simulink model "ITSC2021_CoupledPathFollowingSim_discrete"  (R2019b)
settings: Solver=FixedStepAuto  StartTime=0.0  StopTime=50  FixedStep=0.01  RelTol=1e-4  EnableMultiTasking=on
values from neighbouring files (symbols this model uses):
  friction_grid_cluster = [frictionGrid_Cluster_table.position_x, frictionGrid_Cluster_table.position_y, frictionGrid_Cluster_table.position_z, frictionGrid_Cluster_table.friction_coefficient]    [ITSC2021_runCoupledPathFollowingSim.m]
  inputTrajectory = inputTrajectory(unique_station_indices,:)    [ITSC2021_runCoupledPathFollowingSim.m]
  road_geometry = [sectionRef_table.east, sectionRef_table.north, sectionRef_table.up, sectionRef_table.grade, sectionRef_table.bank, road_geometry_radius, sectionRef_table.yaw]    [ITSC2021_runCoupledPathFollowingSim.m]
undefined symbols (not defined in the file or in its folder): DiscIntNeverNeededParam, flag, initial, mdlparam, mdlParam
libraries: simulink x6, autolibshared x1
(part 3 of 3)

== matlab function ITSC2021_CoupledPathFollowingSim_discrete/Subsystem/ST Friction DB Query/MATLAB Function1 ==
  data: y output; time input
% Purpose: calculate some friction data
% input: time
%
% ouput: friction data of 4 wheels

function y = fric_generator_uml_trip4_vehicleid5010(time)

% Initialization
%A persistent variable is a local variable in a MATLAB function that retains
% its value in memory between calls to the function.
% For code generation, functions must initialize a persistent variable if it is empty.
if time< 150
    y = 0.95*ones(4,1);
elseif time>= 150 && time< 250
    y = 0.85*ones(4,1);
elseif time>= 250 && time< 500
    y = 0.95*ones(4,1);
elseif time>= 500 && time< 600
    y = 0.75*ones(4,1);
elseif time>= 600 && time< 750
    y = 0.9*ones(4,1);
elseif time>= 750 && time< 900
    y = 0.65*ones(4,1);
elseif time>= 900 && time< 1050
    y = 0.85*ones(4,1);
elseif time>= 1050 && time< 1150
    y = 0.55*ones(4,1);
elseif time>= 1150 && time< 1300
    y = 0.85*ones(4,1);
elseif time>= 1300 && time< 1400
    y = 0.45*ones(4,1);
elseif time>= 1400 && time< 1550
    y = 0.75*ones(4,1);
elseif time>= 1550 && time< 1650
    y = 0.35*ones(4,1);
elseif time>= 1650 && time< 1800
    y = 0.85*ones(4,1);
elseif time>= 1800 && time< 2800   
    y = (0.6+0.15*sin(time*2*pi/200))*ones(4,1);
elseif time>= 2800 && time< 2900 
    y = 0.75*ones(4,1);
else
    y = (0.85+0.15*sin(time*2*pi/200))*ones(4,1);
    
end
